simulink model "Rocket_test"  (R2019b)
settings: Solver=VariableStepAuto  StartTime=0  StopTime=100  FixedStep=0.001  MinStep=0.01  RelTol=1e-3
InitFcn:
  | initScript
undefined symbols (not defined in the file): aeng, Anoz, C_IE0, C_LE, cg_rocket, cg_total, Earth, J_rocket, J_total, K1_pitch, l_1st_stage, m_1st_stage_fuel, m_rocket, Omega_earth, Omega_I, P_pvp1, P_pvp2, P_pvp3, P_pvp4, r0, r_1st_stage, sim_dcm, traj_pitch, traj_t, traj_thrust, WGS84, x0, x_1st_stage
libraries: vrlib x9, sharedtransform x4, aerolibtransform2 x1, aerolibasang x1
settings Model: Creator=frizzer  LastModifiedBy=frizzer
settings SolverCC: ZeroCrossAlgorithm=Adaptive
settings DebuggingCC: IgnoredZcDiagnostic=none

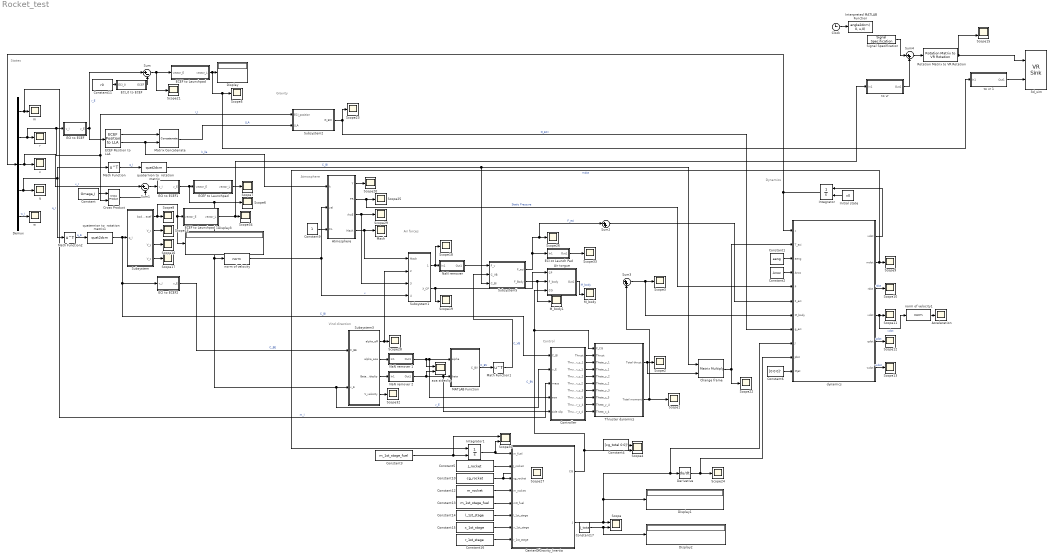
== system Rocket_test ==
  note: Dynamics
  note: Control
  note: Air forces
  note: Gravity
  note: States
  note: Atmosphere
  note: Vind direction
  "3d_sim " : vrlib/VR Sink  InstantiateOnLoad=on  SampleTime=0.1  ViewEnable=on  RemoteChange=off  RemoteView=on  FieldsWritten=Rocket.rotation.4.1.1.double#Rocket.translation.3.1.1.double  WorldFileName=rocket_test_vr.wrl  AutoView=off  VideoDimensions=[200 320]  AllowVariableSize=off  FigureProperties="{'Position', 'Name', 'Viewpoint', 'CameraBound', 'CameraDirection', 'CameraPosition', 'CameraUpVector', 'ZoomFactor', 'Antialiasing', 'Headlight', 'Lighting', 'NavPanel', 'Sound', 'StatusBar', 'Stereo3D', 'Stereo3DCameraOffset', 'Stereo3DHIT', 'ToolBar', 'Textures', 'Transparency', 'Triad', 'Wireframe', 'NavZones', 'NavMode', 'NavSpeed', 'CaptureFileFormat', 'CaptureFileName', 'Record2DCompressMethod', 'Record2DCompressQuality', 'Record2D', 'Record2DFileName', 'Record2DFPS'; [3.0850000000000000e+03   4.9600000000000000e+02   5.7600000000000000e+02   4.2900000000000000e+02], '', 'Rocket', 'on', [3.2020231009351967e-02   9.8606975468551894e-01  -1.6322114967293791e-01], [-4.4051406459118809e+01  -2.7334109397810590e+02  -6.6486808345328058e+01], [9.9894652123826644e-01  -3.6944163507175866e-02  -2.7220883319652722e-02], [1.0000000000000000e+00], 'off', 'on', 'on', 'halfbar', 'on', 'on', 'off', [1.0000000149011612e-01], [0.0000000000000000e+00], 'on', 'on', 'on', 'none', 'off', 'on', 'fly', 'veryslow', 'tif', '%f_anim_%n.tif', 'auto', [7.5000000000000000e+01], 'on', '%f_anim_%n.avi', 'auto'; [3.0000000000000000e+01   6.0000000000000000e+01   3.2000000000000000e+02   2.0000000000000000e+02], '', '', 'on', [0.0000000000000000e+00   0.0000000000000000e+00  -1.0000000000000000e+00], [0.0000000000000000e+00   0.0000000000000000e+00   7.2746134948730457e+01], [0.0000000000000000e+00   1.0000000000000000e+00   0.0000000000000000e+00], [1.0000000000000000e+00], 'on', 'on', 'on', 'none', 'on', 'off', 'off', [1.0000000149011612e-01], [0.0000000000000000e+00], 'off', 'on', 'on', 'none', 'off', 'off', 'fly', 'normal', 'tif', '%f_anim_%n.tif', 'auto', [7.5000000000000000e+01], 'off', '***video***', 'auto'}"
      settings: SourceProductName=Simulink
  "Acceleration " : Scope
  Air torgue : Subsystem
  Atmosphere : MATLAB Function  TreatAsAtomicUnit=on
  CenterOfGravity_Inertia : MATLAB Function  TreatAsAtomicUnit=on
  Change frame : Product  Multiplication=Matrix(*)
  Clock : Clock
  Constant : Constant  Value=Omega_I
  Constant1 : Constant  Value=aeng
  Constant10 : Constant  Value=cg_rocket
  Constant11 : Constant  Value=r0
  Constant12 : Constant  Value=m_rocket
  Constant13 : Constant  Value=m_1st_stage_fuel
  Constant14 : Constant  Value=l_1st_stage
  Constant15 : Constant  Value=x_1st_stage
  Constant16 : Constant  Value=r_1st_stage
  Constant17 : Constant  Value=J_total
  Constant2 : Constant  Value=Anoz
  Constant3 : Constant  Value=m_1st_stage_fuel
  Constant4 : Constant  Value=[cg_total 0 0]'
  Constant5 : Constant  Value=J_rocket
  Constant6 : Constant  Value=[0 0 0]'
  Constant9 : Constant
  Controller : Subsystem
  Cross Product : vrlib/Utilities/Cross Product
      settings: SourceProductName=Simulink
  Demux : Demux  Outputs=[1 3 3 4 3]
  Derivative : Derivative
  Display{,1..3} (4 alike) : Display
      Display settings: Decimation=6
      Display1 settings: Decimation=6
      Display2 settings: Decimation=6
  "ECEF Position to LLA " : aerolibtransform2/ECEF Position to LLA  units=Metric (MKS)  ptype=Earth (WGS84)  F=1/298.257223563  R=6378137
      settings: SourceProductName=Aerospace Blockset  SourceProductBaseCode=AE
  ECEF to Launchpad : Subsystem
  "ECEF to Launchpad " : Subsystem
  ECEF to Launchpad 1 : Subsystem
  ECI ot Launch Pad : Subsystem
  ECI to ECEF : Subsystem
  ECI to ECEF1 : Subsystem
  ECI to ECEF2 : Subsystem
  ECI_0 to ECEF : Subsystem
  Initial state : Constant  Value=x0
  Integrator : Integrator  InitialConditionSource=external  InitialCondition=x0
  Integrator1 : Integrator  InitialConditionSource=external  InitialCondition=x0
  Interpreted MATLAB Function : MATLABFcn  MATLABFcn=angle2dcm( 0, u,0)
  MATLAB Function : MATLAB Function  TreatAsAtomicUnit=on
  M_body : Scope
  M_body1 : Scope
  "Mach " : Scope
  Math Function : Math  Operator=transpose  SignedPower=off  SaturateOnIntegerOverflow=on
  Math Function1 : Math  Operator=transpose  SignedPower=off  SaturateOnIntegerOverflow=on
  Math Function2 : Math  Operator=transpose  SignedPower=off  SaturateOnIntegerOverflow=on
  Matrix Concatenate : Concatenate  ConcatenateDimension=3
  "NaN remover " : Subsystem
  NaN remover 1 : Subsystem
  NaN remover 2 : Subsystem
  Rotation Matrix to VR Rotation : vrlib/Utilities/Rotation Matrix to VR Rotation  maxzero=1e-12
      settings: SourceProductName=Simulink  SourceProductBaseCode=SL
  Scope{,4,15,30} (4 alike) : Scope  NumInputPorts=2
  Scope{1..3,5..14,16..29,32..34} (30 alike) : Scope
  Signal Specification : SignalSpecification  Dimensions=[3 3]
  Subsystem : Subsystem
  Subsystem1 : Subsystem
  Subsystem2 : Subsystem
  Subsystem3 : Subsystem
  Subsystem5 : Subsystem
  Sum : Sum  Inputs=|+-
  Sum1 : Sum  Inputs=|+-
  Sum2 : Sum  Inputs=|++
  Sum3 : Sum  Inputs=|++
  Sum4 : Sum  Inputs=|++
  Thruster dynamics : Subsystem
  "aoa sideslip " : Scope  NumInputPorts=2
  dynamics : MATLAB Function  TreatAsAtomicUnit=on
  m : Scope
  norm of velocity : MATLABFcn  MATLABFcn=norm  Output1D=off
  norm of velocity1 : MATLABFcn  MATLABFcn=norm  Output1D=off
  q : Scope
  quaternion to  rotation matrix : MATLABFcn  MATLABFcn=quat2dcm  Output1D=off
  quaternion to  rotation matrix1 : MATLABFcn  MATLABFcn=quat2dcm  Output1D=off
  r : Scope
  "to vr " : Subsystem
  to vr 1 : Subsystem
  v : Scope
  w : Scope
  wires:
  Initial state/1 -> Integrator/2
  Constant1/1 -> dynamics/3(aeng)
  ECEF to Launchpad/1(vector_L) -> Scope7/1
  dynamics/1(xdot) -> Integrator/1
  Sum2/1 -> dynamics/6(F_eci)
  Derivative/1 -> dynamics/10(Jdot), Scope24/1
  Constant11/1 -> ECI_0 to ECEF/1(ECI_0)
  Constant2/1 -> dynamics/4(Anoz)
  Constant/1 -> Cross Product/1
  dynamics/3(rdot) -> Scope10/1  "rdot"
  quaternion to  rotation matrix/1 -> Change frame/1, Subsystem5/3(C_BI)  "C_BI"
  Cross Product/1 -> Sum1/2
  dynamics/5(qdot) -> Scope12/1  "qdot"
  ECI to ECEF1/1(v_E) -> Controller/2(v_E), Subsystem3/2(v_E), norm of velocity/1, Scope6/1, ECEF to Launchpad/1("vector_E ")  "v_E"
  Subsystem5/1(F_eci) -> Sum2/1, Scope26/1, ECI ot Launch Pad/1(In1)  "F_eci"
  Sum1/1 -> ECI to ECEF1/1("v_I ")
  dynamics/6(wdot) -> Scope13/1  "wdot"
  ECI_0 to ECEF/1(ECEF) -> Sum/2
  Constant6/1 -> dynamics/11(Mjet)
  Subsystem/1(body in ecef) -> Display3/1, ECEF to Launchpad 1/1("vector_E "), Scope8/1
  dynamics/2(mdot) -> Integrator1/1, Scope9/1  "mdot"
  Math Function/1 -> quaternion to  rotation matrix/1  "q_I"
  Atmosphere/1(Y) -> Scope20/1
  Subsystem/4(V_z) -> Scope17/1
  Subsystem3/1(alpha_eff) -> Subsystem1/2(alpha_eff), Scope28/1
  ECI to ECEF2/1(v_E) -> Subsystem3/1(C_BE)  "C_BE"
  Subsystem3/4(V_velocity) -> Scope32/1
  Demux/4 -> q/1, Math Function/1, Math Function2/1  "q_I"
  Constant9/1 -> Atmosphere/3(CL)
  Subsystem3/2(alpha_aoa) -> NaN remover 1/1(In1)
  ECI ot Launch Pad/1(Out1) -> Scope33/1
  MATLAB Function/1(C_BV) -> Math Function1/1  "C_BV"
  Subsystem1/2("X_CP ") -> Scope19/1, Air torgue/1(CP)
  norm of velocity1/1 -> "Acceleration "/1
  Sum3/1 -> Scope3/1, dynamics/7(M_body)
  Atmosphere/3(rhoE) -> Subsystem1/3(air_density), Scope29/1
  Math Function1/1 -> Subsystem5/2(C_VB)  "C_VB"
  Air torgue/1(Out1) -> M_body/1  "M_body"
  Subsystem5/2(F_Body) -> M_body1/1, Air torgue/2(F_body)
  Subsystem3/3(Beta_sideslip) -> NaN remover 2/1(In1)
  Thruster dynamics/1(Total thrust) -> Change frame/2, Scope2/1
  quaternion to  rotation matrix1/1 -> ECI to ECEF2/1("v_I "), Controller/1(C_BI), Subsystem/1(q_I)  "C_BI"
  NaN remover 1/1(Out1) -> "aoa sideslip "/1, MATLAB Function/1(alpha), Controller/4(aoa)
  Change frame/1 -> dynamics/2(T_eci), Scope22/1
  Demux/1 -> Controller/3(mass), m/1  "m_I"
  Integrator/1 -> Demux/1, dynamics/1(x)
  CenterOfGravity_Inertia/2(J) -> Scope/1, dynamics/9(J), Derivative/1, Display1/1
  Atmosphere/2(PR) -> dynamics/5(P), Scope25/1  "Static Pressure"
  norm of velocity/1 -> Atmosphere/2(vel), Subsystem1/4(air_speed)  "v"
  Atmosphere/4(Mach) -> Subsystem1/1(Mach), "Mach "/1
  Subsystem1/1(F_aero) -> Scope18/1, "NaN remover "/1(In1)
  NaN remover 2/1(Out1) -> Controller/5(side slip), MATLAB Function/2(beta), "aoa sideslip "/2
  Thruster dynamics/2(Total moment) -> Sum3/2, Scope1/1
  Subsystem/2(V_x) -> Scope14/1
  dynamics/4(vdot) -> norm of velocity1/1, Scope11/1  "vdot"
  Matrix Concatenate/1 -> Subsystem2/2("LLA ")  "LLA"
  "NaN remover "/1(Out1) -> Subsystem5/1(F_v)
  Demux/5 -> w/1  "w_I"
  Math Function2/1 -> quaternion to  rotation matrix1/1  "q_E"
  Subsystem/3(V_y) -> Scope16/1
  "ECEF Position to LLA "/1 -> Matrix Concatenate/1
  Demux/2 -> r/1, Subsystem2/1(ECI_position), Cross Product/2, ECI to ECEF/1("v_I ")  "r_I"
  Demux/3 -> v/1, Sum1/1  "v_I"
  ECI to ECEF/1(v_E) -> "ECEF Position to LLA "/1, Sum/1  "r_E"
  "ECEF to Launchpad "/1(vector_L) -> to vr 1/1(In1), Scope5/1, Display/1
  Sum/1 -> "ECEF to Launchpad "/1("vector_E "), Scope21/1
  Subsystem2/1(G_ECI) -> Scope23/1, dynamics/8(g_eci)  "G_ECI"
  "ECEF Position to LLA "/2 -> Atmosphere/1(h), Matrix Concatenate/2  "h_lla"
  Constant3/1 -> Scope30/1, Integrator1/2
  Constant5/1 -> CenterOfGravity_Inertia/2(J_rocket)
  Constant10/1 -> Scope27/1, CenterOfGravity_Inertia/3(cg_rocket)
  Constant12/1 -> CenterOfGravity_Inertia/4(m_rocket)
  Constant13/1 -> CenterOfGravity_Inertia/5(m0_fuel)
  Constant14/1 -> CenterOfGravity_Inertia/6(l_1st_stage)
  Constant15/1 -> CenterOfGravity_Inertia/7(x_1st_stage)
  Constant16/1 -> CenterOfGravity_Inertia/8(r_1st_stage)
  CenterOfGravity_Inertia/1(CG) -> Thruster dynamics/1(P_CG), Air torgue/3(CG), Scope4/2  "C_BV"
  Constant17/1 -> Display2/1, Scope/2
  Integrator1/1 -> Scope30/2, CenterOfGravity_Inertia/1(m_fuel)
  Constant4/1 -> Scope4/1
  Controller/1(Thrust) -> Thruster dynamics/2(Thrust)
  Controller/2(Thruster_y_1) -> Thruster dynamics/3(Theta_y_1)
  Controller/3(Thruster_z_1) -> Thruster dynamics/4(Theta_z_1)
  Controller/4(Thruster_y_2) -> Thruster dynamics/5(Theta_y_2)
  Controller/5(Thruster_z_2) -> Thruster dynamics/6(Theta_z_2)
  Controller/6(Thruster_y_3) -> Thruster dynamics/7(Theta_y_3)
  Controller/7(Thruster_z_3) -> Thruster dynamics/8(Theta_z_3)
  Controller/8(Thruster_y_4) -> Thruster dynamics/9(Theta_y_4)
  Controller/9(Thruster_z_4) -> Thruster dynamics/10(Theta_z_4)
  Clock/1 -> Interpreted MATLAB Function/1
  Rotation Matrix to VR Rotation/1 -> Scope15/2, "3d_sim "/1
  ECEF to Launchpad 1/1(vector_L) -> "to vr "/1(In1), Scope34/1
  Signal Specification/1 -> Sum4/1
  Sum4/1 -> Rotation Matrix to VR Rotation/1
  "to vr "/1(Out1) -> Sum4/2
  to vr 1/1(Out1) -> "3d_sim "/2

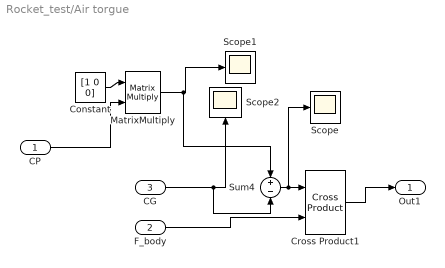
== system Rocket_test/Air torgue ==
  CP : Inport
  F_body : Inport  Port=2
  CG : Inport  Port=3
  Constant : Constant  Value=[1 0 0]
  Cross Product1 : vrlib/Utilities/Cross Product
      settings: SourceProductName=Simulink
  MatrixMultiply : Product  Multiplication=Matrix(*)
  Scope : Scope
  Scope1 : Scope
  Scope2 : Scope
  Sum4 : Sum  Inputs=+-
  Out1 : Outport
  wires:
  CP/1 -> MatrixMultiply/2
  Sum4/1 -> Scope/1, Cross Product1/1
  CG/1 -> Scope2/1, Sum4/2
  F_body/1 -> Cross Product1/2
  Cross Product1/1 -> Out1/1
  Constant/1 -> MatrixMultiply/1
  MatrixMultiply/1 -> Sum4/1, Scope1/1

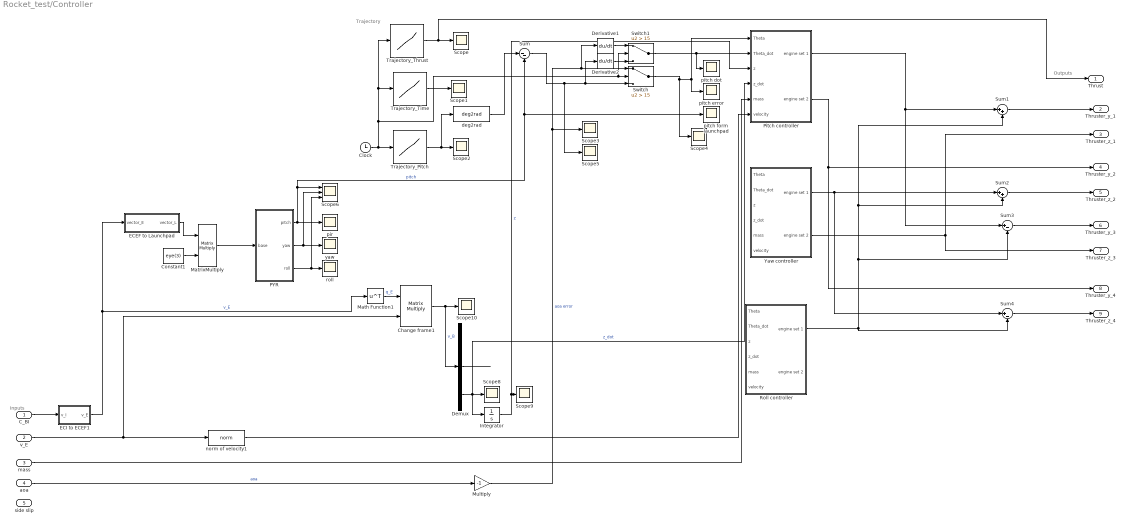
== system Rocket_test/Controller ==
  note: Inputs
  note: Trajectory
  note: Outputs
  C_BI : Inport
  v_E : Inport  Port=2
  mass : Inport  Port=3
  aoa : Inport  Port=4
  side slip : Inport  Port=5
  Change frame1 : Product  Multiplication=Matrix(*)
  Clock : Clock
  Constant1 : Constant  Value=eye(3)
  Demux : Demux  Outputs=3
  Derivative1 : Derivative
  Derivative2 : Derivative
  ECEF to Launchpad : Subsystem
  ECI to ECEF1 : Subsystem
  Integrator : Integrator
  Math Function1 : Math  Operator=transpose  SignedPower=off  SaturateOnIntegerOverflow=on
  MatrixMultiply : Product  Multiplication=Matrix(*)
  Multiply : Gain  Gain=-1
  PYR : MATLAB Function  TreatAsAtomicUnit=on
  Pitch controller : Subsystem
  Roll controller : Subsystem
  Scope{,1..5,8..10} (9 alike) : Scope
  Scope6 : Scope  NumInputPorts=3
  Sum : Sum  Inputs=|--
  Sum1 : Sum  Inputs=|++
  Sum2 : Sum  Inputs=|++
  Sum3 : Sum  Inputs=|+-
  Sum4 : Sum  Inputs=|+-
  Switch : Switch  Criteria=u2 > Threshold  Threshold=15
  Switch1 : Switch  Criteria=u2 > Threshold  Threshold=15
  Trajectory_Pitch : Lookup_n-D  NumberOfTableDimensions=1  BreakpointsForDimension1=traj_t  Table=traj_pitch  InternalRulePriority=Speed  RndMeth=Simplest  InputSameDT=on
  Trajectory_Thrust : Lookup_n-D  NumberOfTableDimensions=1  BreakpointsForDimension1=traj_t  Table=traj_thrust  InternalRulePriority=Speed  RndMeth=Simplest  InputSameDT=on
  Trajectory_Time : Lookup_n-D  NumberOfTableDimensions=1  BreakpointsForDimension1=traj_t  Table=traj_t  InternalRulePriority=Speed  RndMeth=Simplest  InputSameDT=on
  Yaw controller : Subsystem
  deg2rad : MATLABFcn  MATLABFcn=deg2rad
  norm of velocity1 : MATLABFcn  MATLABFcn=norm  Output1D=off
  pir : Scope
  pitch dot : Scope
  pitch error : Scope
  pitch form launchpad : Scope
  "roll " : Scope
  yaw : Scope
  Thrust : Outport
  Thruster_y_1 : Outport  Port=2
  Thruster_z_1 : Outport  Port=3
  Thruster_y_2 : Outport  Port=4
  Thruster_z_2 : Outport  Port=5
  Thruster_y_3 : Outport  Port=6
  Thruster_z_3 : Outport  Port=7
  Thruster_y_4 : Outport  Port=8
  Thruster_z_4 : Outport  Port=9
  wires:
  v_E/1 -> norm of velocity1/1, Change frame1/2
  norm of velocity1/1 -> Pitch controller/6(velocity)
  Change frame1/1 -> Scope10/1, Demux/1  "v_B"
  Math Function1/1 -> Change frame1/1  "q_E"
  deg2rad/1 -> Sum/1
  Roll controller/1(engine set 1) -> Sum4/2, Sum2/2, Sum1/2, Sum3/2
  MatrixMultiply/1 -> PYR/1(base)
  Yaw controller/1(engine set 1) -> Sum4/1, Sum2/1
  Sum4/1 -> Thruster_z_4/1
  C_BI/1 -> ECI to ECEF1/1("v_I ")
  Switch1/1 -> Pitch controller/2(Theta_dot), pitch dot/1
  Integrator/1 -> Pitch controller/3(z), Scope9/1  "z"
  Demux/3 -> Pitch controller/4(z_dot), Scope8/1, Integrator/1  "z_dot"
  Yaw controller/2(engine set 2) -> Thruster_z_3/1, Thruster_z_1/1
  Trajectory_Pitch/1 -> deg2rad/1, Scope2/1
  Pitch controller/1(engine set 1) -> Sum3/1, Sum1/1
  PYR/1(pitch) -> Sum/2, pitch form launchpad/1, Scope6/1, pir/1  "pitch"
  Sum3/1 -> Thruster_y_3/1
  Pitch controller/2(engine set 2) -> Thruster_y_4/1, Thruster_y_2/1
  ECI to ECEF1/1(v_E) -> ECEF to Launchpad/1("vector_E "), Math Function1/1  "v_E"
  mass/1 -> Pitch controller/5(mass)
  Clock/1 -> Switch1/2, Switch/2, Trajectory_Time/1, Trajectory_Thrust/1, Trajectory_Pitch/1
  PYR/2(yaw) -> yaw/1, Scope6/2
  ECEF to Launchpad/1(vector_L) -> MatrixMultiply/1
  Trajectory_Thrust/1 -> Thrust/1, Scope/1
  Constant1/1 -> MatrixMultiply/2
  PYR/3(roll) -> Scope6/3, "roll "/1
  Trajectory_Time/1 -> Scope1/1
  Sum2/1 -> Thruster_z_2/1
  Sum1/1 -> Thruster_y_1/1
  Demux/2 -> ?
  aoa/1 -> Multiply/1  "aoa"
  Sum/1 -> Scope5/1, Derivative2/1, Switch/3
  Switch/1 -> Pitch controller/1(Theta), pitch error/1, Scope4/1
  Derivative1/1 -> Switch1/1
  Derivative2/1 -> Switch1/3
  Multiply/1 -> Scope3/1, Derivative1/1, Switch/1  "aoa error"

== system Rocket_test/ECEF to Launchpad ==
  "vector_E " : Inport
  Change frame2 : Product  Multiplication=Matrix(*)
  ECEF to L 2 : Constant  Value=C_LE
  Math Function1 : Math  Operator=transpose  SignedPower=off  SaturateOnIntegerOverflow=on
  vector_L : Outport
  wires:
  "vector_E "/1 -> Change frame2/2
  ECEF to L 2/1 -> Math Function1/1
  Change frame2/1 -> vector_L/1
  Math Function1/1 -> Change frame2/1

== system Rocket_test/ECEF to Launchpad  ==
  "vector_E " : Inport
  Change frame2 : Product  Multiplication=Matrix(*)
  ECEF to L 2 : Constant  Value=C_LE
  Math Function1 : Math  Operator=transpose  SignedPower=off  SaturateOnIntegerOverflow=on
  vector_L : Outport
  wires:
  "vector_E "/1 -> Change frame2/2
  ECEF to L 2/1 -> Math Function1/1
  Change frame2/1 -> vector_L/1
  Math Function1/1 -> Change frame2/1

== system Rocket_test/ECEF to Launchpad 1 ==
  "vector_E " : Inport
  Change frame2 : Product  Multiplication=Matrix(*)
  ECEF to L 2 : Constant  Value=C_LE
  Math Function1 : Math  Operator=transpose  SignedPower=off  SaturateOnIntegerOverflow=on
  vector_L : Outport
  wires:
  "vector_E "/1 -> Change frame2/2
  ECEF to L 2/1 -> Math Function1/1
  Change frame2/1 -> vector_L/1
  Math Function1/1 -> Change frame2/1

== system Rocket_test/ECI ot Launch Pad ==
  In1 : Inport
  ECEF to Launchpad 1 : Subsystem
  ECI to ECEF4 : Subsystem
  Out1 : Outport
  wires:
  ECI to ECEF4/1(v_E) -> ECEF to Launchpad 1/1("vector_E ")
  ECEF to Launchpad 1/1(vector_L) -> Out1/1
  In1/1 -> ECI to ECEF4/1("v_I ")

== system Rocket_test/ECI to ECEF ==
  "v_I " : Inport
  Change frame2 : Product  Inputs=3  Multiplication=Matrix(*)
  Clock1 : Clock
  Constant1 : Constant  Value=Omega_earth
  ECEF to L 2 : Constant  Value=C_IE0
  MATLAB Function1 : MATLAB Function  TreatAsAtomicUnit=on
  v_E : Outport
  wires:
  MATLAB Function1/1(C_IE_t) -> Change frame2/1
  "v_I "/1 -> Change frame2/3
  Constant1/1 -> MATLAB Function1/2(Omega_earth)
  Clock1/1 -> MATLAB Function1/1(t)
  Change frame2/1 -> v_E/1
  ECEF to L 2/1 -> Change frame2/2

== system Rocket_test/ECI to ECEF1 ==
  "v_I " : Inport
  Change frame2 : Product  Inputs=3  Multiplication=Matrix(*)
  Clock1 : Clock
  Constant1 : Constant  Value=Omega_earth
  ECEF to L 2 : Constant  Value=C_IE0
  MATLAB Function1 : MATLAB Function  TreatAsAtomicUnit=on
  v_E : Outport
  wires:
  MATLAB Function1/1(C_IE_t) -> Change frame2/1
  "v_I "/1 -> Change frame2/3
  Constant1/1 -> MATLAB Function1/2(Omega_earth)
  Clock1/1 -> MATLAB Function1/1(t)
  Change frame2/1 -> v_E/1
  ECEF to L 2/1 -> Change frame2/2

== system Rocket_test/ECI to ECEF2 ==
  "v_I " : Inport
  Change frame2 : Product  Inputs=3  Multiplication=Matrix(*)
  Clock1 : Clock
  Constant1 : Constant  Value=Omega_earth
  ECEF to L 2 : Constant  Value=C_IE0
  MATLAB Function1 : MATLAB Function  TreatAsAtomicUnit=on
  v_E : Outport
  wires:
  ECEF to L 2/1 -> Change frame2/2
  Change frame2/1 -> v_E/1
  Clock1/1 -> MATLAB Function1/1(t)
  Constant1/1 -> MATLAB Function1/2(Omega_earth)
  "v_I "/1 -> Change frame2/3
  MATLAB Function1/1(C_IE_t) -> Change frame2/1

== system Rocket_test/ECI_0 to ECEF ==
  ECI_0 : Inport
  Constant12 : Constant  Value=C_IE0
  MatrixMultiply : Product  Multiplication=Matrix(*)
  ECEF : Outport
  wires:
  Constant12/1 -> MatrixMultiply/1
  MatrixMultiply/1 -> ECEF/1
  ECI_0/1 -> MatrixMultiply/2

== system Rocket_test/NaN remover  ==
  In1 : Inport
  Constant4 : Constant  Value=[0 0 0]'
  IsNaN : RelationalOperator  Operator=isNaN  OutDataTypeStr=boolean  RndMeth=Simplest
  "NaN " : Scope
  Switch : Switch  Criteria=u2 > Threshold
  Out1 : Outport
  wires:
  IsNaN/1 -> "NaN "/1, Switch/2
  Constant4/1 -> Switch/1
  In1/1 -> IsNaN/1, Switch/3
  Switch/1 -> Out1/1

== system Rocket_test/NaN remover 1 ==
  In1 : Inport
  Constant4 : Constant  Value=0
  IsNaN : RelationalOperator  Operator=isNaN  OutDataTypeStr=boolean  RndMeth=Simplest
  "NaN " : Scope
  Switch : Switch  Criteria=u2 > Threshold
  Out1 : Outport
  wires:
  Switch/1 -> Out1/1
  In1/1 -> Switch/3, IsNaN/1
  Constant4/1 -> Switch/1
  IsNaN/1 -> Switch/2, "NaN "/1

== system Rocket_test/NaN remover 2 ==
  In1 : Inport
  Constant4 : Constant  Value=0
  IsNaN : RelationalOperator  Operator=isNaN  OutDataTypeStr=boolean  RndMeth=Simplest
  "NaN " : Scope
  Switch : Switch  Criteria=u2 > Threshold
  Out1 : Outport
  wires:
  IsNaN/1 -> "NaN "/1, Switch/2
  Constant4/1 -> Switch/1
  In1/1 -> IsNaN/1, Switch/3
  Switch/1 -> Out1/1

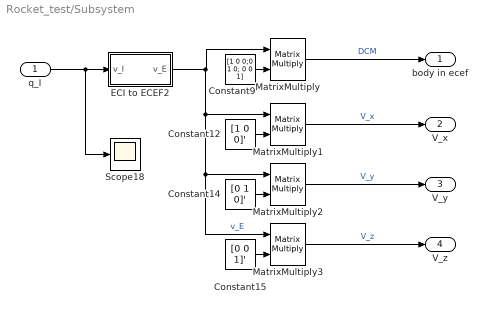
== system Rocket_test/Subsystem ==
  q_I : Inport
  Constant12 : Constant  Value=[1 0 0]'
  Constant14 : Constant  Value=[0 1 0]'
  Constant15 : Constant  Value=[0 0 1]'
  Constant9 : Constant  Value=[1 0 0;0 1 0; 0 0 1]
  ECI to ECEF2 : Subsystem
  MatrixMultiply{,1..3} (4 alike) : Product  Multiplication=Matrix(*)
  Scope18 : Scope
  body in ecef : Outport
  V_x : Outport  Port=2
  V_y : Outport  Port=3
  V_z : Outport  Port=4
  wires:
  MatrixMultiply/1 -> body in ecef/1  "DCM"
  ECI to ECEF2/1(v_E) -> MatrixMultiply3/1, MatrixMultiply2/1, MatrixMultiply1/1, MatrixMultiply/1  "v_E"
  q_I/1 -> Scope18/1, ECI to ECEF2/1("v_I ")
  Constant9/1 -> MatrixMultiply/2
  Constant14/1 -> MatrixMultiply2/2
  Constant12/1 -> MatrixMultiply1/2
  MatrixMultiply1/1 -> V_x/1  "V_x"
  Constant15/1 -> MatrixMultiply3/2
  MatrixMultiply2/1 -> V_y/1  "V_y"
  MatrixMultiply3/1 -> V_z/1  "V_z"

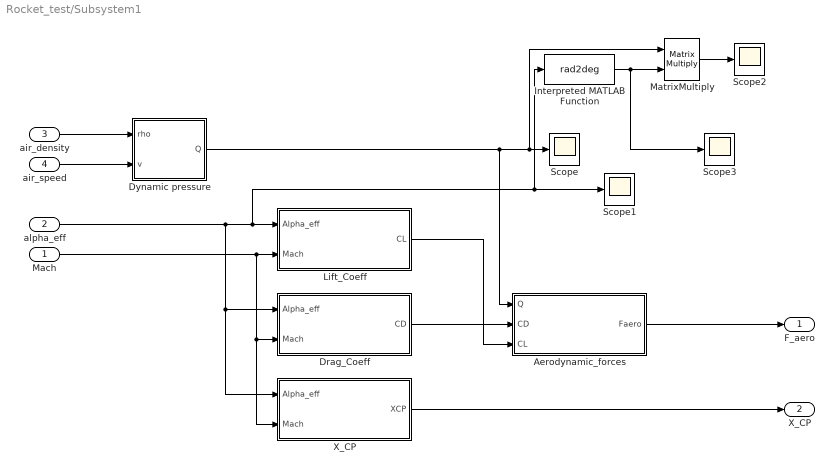
== system Rocket_test/Subsystem1 ==
  Mach : Inport
  alpha_eff : Inport  Port=2
  air_density : Inport  Port=3
  air_speed : Inport  Port=4
  Aerodynamic_forces : MATLAB Function  TreatAsAtomicUnit=on
  Drag_Coeff : MATLAB Function  TreatAsAtomicUnit=on
  Dynamic pressure : MATLAB Function  TreatAsAtomicUnit=on
  Interpreted MATLAB Function : MATLABFcn  MATLABFcn=rad2deg
  Lift_Coeff : MATLAB Function  TreatAsAtomicUnit=on
  MatrixMultiply : Product  Multiplication=Matrix(*)
  Scope{,1..3} (4 alike) : Scope
  X_CP : MATLAB Function  TreatAsAtomicUnit=on
  F_aero : Outport
  "X_CP " : Outport  Port=2
  wires:
  air_density/1 -> Dynamic pressure/1(rho)
  X_CP/1(XCP) -> "X_CP "/1
  Mach/1 -> X_CP/2(Mach), Drag_Coeff/2(Mach), Lift_Coeff/2(Mach)
  Lift_Coeff/1(CL) -> Aerodynamic_forces/3(CL)
  Drag_Coeff/1(CD) -> Aerodynamic_forces/2(CD)
  Aerodynamic_forces/1(Faero) -> F_aero/1
  alpha_eff/1 -> X_CP/1(Alpha_eff), Drag_Coeff/1(Alpha_eff), Interpreted MATLAB Function/1, Scope1/1, Lift_Coeff/1(Alpha_eff)
  Dynamic pressure/1(Q) -> MatrixMultiply/1, Scope/1, Aerodynamic_forces/1(Q)
  air_speed/1 -> Dynamic pressure/2(v)
  MatrixMultiply/1 -> Scope2/1
  Interpreted MATLAB Function/1 -> Scope3/1, MatrixMultiply/2

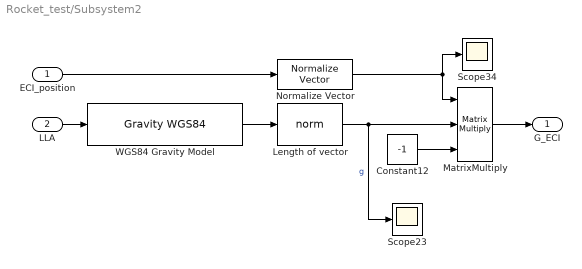
== system Rocket_test/Subsystem2 ==
  ECI_position : Inport
  "LLA " : Inport  Port=2
  Constant12 : Constant  Value=-1
  Length of vector : MATLABFcn  MATLABFcn=norm  Output1D=off
  MatrixMultiply : Product  Inputs=3  Multiplication=Matrix(*)
  Normalize Vector : vrlib/Utilities/Normalize Vector  maxzero=0
      settings: SourceProductName=Simulink
  Scope23 : Scope
  Scope34 : Scope
  "WGS84 Gravity Model  " : GravityWGS84  BlockKeywords=__PRM__SERIALIZED__DATA__:world geodetic system,WGS 84,geocentric,equipotential,ellipsoid,WGS84 taylor series,WGS84 close approximation,WGS84 exact,Earth,1984,Earth gravity,planetary gravity,gravitational field
  G_ECI : Outport
  wires:
  Length of vector/1 -> Scope23/1, MatrixMultiply/2  "g"
  Normalize Vector/1 -> MatrixMultiply/1, Scope34/1
  MatrixMultiply/1 -> G_ECI/1
  "WGS84 Gravity Model  "/1 -> Length of vector/1
  Constant12/1 -> MatrixMultiply/3
  "LLA "/1 -> "WGS84 Gravity Model  "/1
  ECI_position/1 -> Normalize Vector/1

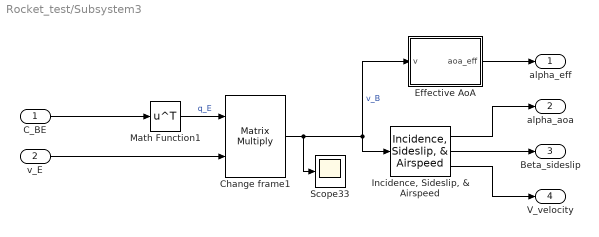
== system Rocket_test/Subsystem3 ==
  C_BE : Inport
  v_E : Inport  Port=2
  Change frame1 : Product  Multiplication=Matrix(*)
  Effective AoA : MATLAB Function  TreatAsAtomicUnit=on
  "Incidence, Sideslip, & Airspeed" : aerolibasang/Incidence, Sideslip, & Airspeed
      settings: SourceProductName=Aerospace Blockset
  Math Function1 : Math  Operator=transpose  SignedPower=off  SaturateOnIntegerOverflow=on
  Scope33 : Scope
  alpha_eff : Outport
  alpha_aoa : Outport  Port=2
  Beta_sideslip : Outport  Port=3
  V_velocity : Outport  Port=4
  wires:
  "Incidence, Sideslip, & Airspeed"/3 -> V_velocity/1
  Math Function1/1 -> Change frame1/1  "q_E"
  Change frame1/1 -> Scope33/1, Effective AoA/1(v), "Incidence, Sideslip, & Airspeed"/1  "v_B"
  C_BE/1 -> Math Function1/1
  Effective AoA/1(aoa_eff) -> alpha_eff/1
  v_E/1 -> Change frame1/2
  "Incidence, Sideslip, & Airspeed"/1 -> alpha_aoa/1
  "Incidence, Sideslip, & Airspeed"/2 -> Beta_sideslip/1

== system Rocket_test/Subsystem5 ==
  F_v : Inport
  C_VB : Inport  Port=2
  C_BI : Inport  Port=3
  MatrixMultiply : Product  Multiplication=Matrix(*)
  MatrixMultiply1 : Product  Multiplication=Matrix(*)
  F_eci : Outport
  F_Body : Outport  Port=2
  wires:
  F_v/1 -> MatrixMultiply/2
  MatrixMultiply/1 -> F_Body/1, MatrixMultiply1/2
  C_VB/1 -> MatrixMultiply/1
  C_BI/1 -> MatrixMultiply1/1
  MatrixMultiply1/1 -> F_eci/1

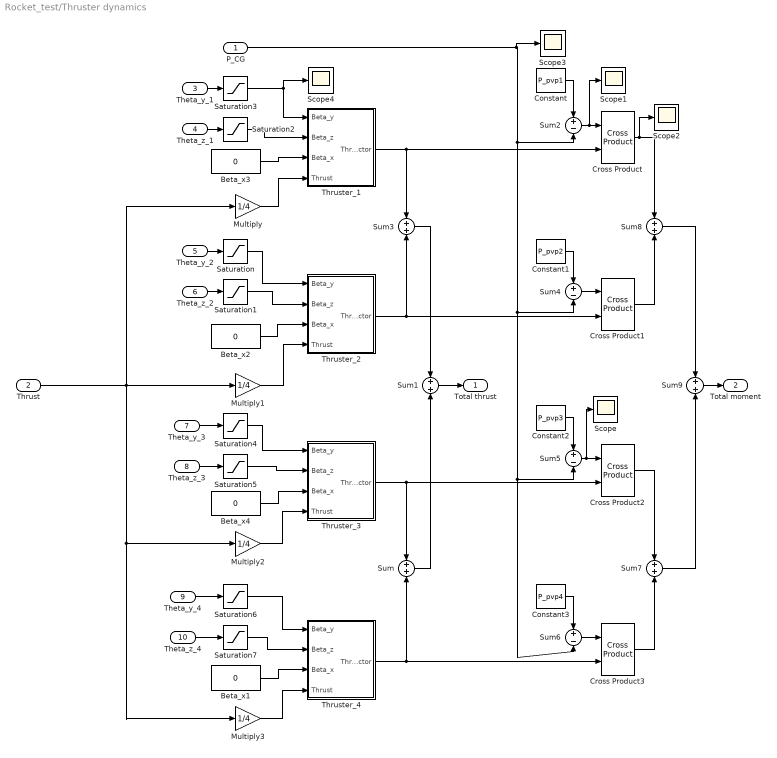
== system Rocket_test/Thruster dynamics ==
  P_CG : Inport
  Thrust : Inport  Port=2
  Theta_y_1 : Inport  Port=3
  Theta_z_1 : Inport  Port=4
  Theta_y_2 : Inport  Port=5
  Theta_z_2 : Inport  Port=6
  Theta_y_3 : Inport  Port=7
  Theta_z_3 : Inport  Port=8
  Theta_y_4 : Inport  Port=9
  Theta_z_4 : Inport  Port=10
  Beta_x{1..4} (4 alike) : Constant  Value=0
  Constant : Constant  Value=P_pvp1
  Constant1 : Constant  Value=P_pvp2
  Constant2 : Constant  Value=P_pvp3
  Constant3 : Constant  Value=P_pvp4
  Cross Product{,1..3} (4 alike) : vrlib/Utilities/Cross Product
      settings: SourceProductName=Simulink
  Multiply{,1..3} (4 alike) : Gain  Gain=1/4
  Saturation : Saturate  UpperLimit=deg2rad(6)  LowerLimit=deg2rad(-6)
  Saturation{1..7} (7 alike) : Saturate  UpperLimit=deg2rad(6)  LowerLimit=deg2rad(-6)  ZeroCross=off
  Scope{,1..4} (5 alike) : Scope
  Sum{,1,3,7..9} (6 alike) : Sum
  Sum{2,4..6} (4 alike) : Sum  Inputs=+-
  Thruster_1 : Subsystem
  Thruster_2 : Subsystem
  Thruster_3 : Subsystem
  Thruster_4 : Subsystem
  Total thrust : Outport
  Total moment : Outport  Port=2
  wires:
  Thrust/1 -> Multiply3/1, Multiply2/1, Multiply1/1, Multiply/1
  Beta_x1/1 -> Thruster_4/3(Beta_x)
  Theta_z_4/1 -> Saturation7/1
  Theta_y_4/1 -> Saturation6/1
  Thruster_4/1(Thrust_vector) -> Sum/2, Cross Product3/2
  Theta_y_3/1 -> Saturation4/1
  Theta_z_3/1 -> Saturation5/1
  Beta_x4/1 -> Thruster_3/3(Beta_x)
  Thruster_3/1(Thrust_vector) -> Cross Product2/2, Sum/1
  Thruster_1/1(Thrust_vector) -> Cross Product/2, Sum3/1
  Beta_x3/1 -> Thruster_1/3(Beta_x)
  Theta_z_1/1 -> Saturation2/1
  Theta_y_1/1 -> Saturation3/1
  Thruster_2/1(Thrust_vector) -> Sum3/2, Cross Product1/2
  Theta_y_2/1 -> Saturation/1
  Theta_z_2/1 -> Saturation1/1
  Beta_x2/1 -> Thruster_2/3(Beta_x)
  Sum3/1 -> Sum1/1
  Sum/1 -> Sum1/2
  Sum1/1 -> Total thrust/1
  P_CG/1 -> Scope3/1, Sum2/2, Sum4/2, Sum5/2, Sum6/2
  Sum2/1 -> Scope1/1, Cross Product/1
  Constant/1 -> Sum2/1
  Constant1/1 -> Sum4/1
  Sum4/1 -> Cross Product1/1
  Sum5/1 -> Scope/1, Cross Product2/1
  Constant2/1 -> Sum5/1
  Constant3/1 -> Sum6/1
  Sum6/1 -> Cross Product3/1
  Cross Product3/1 -> Sum7/2
  Cross Product2/1 -> Sum7/1
  Cross Product1/1 -> Sum8/2
  Cross Product/1 -> Scope2/1, Sum8/1
  Sum8/1 -> Sum9/1
  Sum7/1 -> Sum9/2
  Sum9/1 -> Total moment/1
  Multiply/1 -> Thruster_1/4(Thrust)
  Multiply1/1 -> Thruster_2/4(Thrust)
  Multiply2/1 -> Thruster_3/4(Thrust)
  Multiply3/1 -> Thruster_4/4(Thrust)
  Saturation/1 -> Thruster_2/1(Beta_y)
  Saturation1/1 -> Thruster_2/2(Beta_z)
  Saturation2/1 -> Thruster_1/2(Beta_z)
  Saturation3/1 -> Scope4/1, Thruster_1/1(Beta_y)
  Saturation4/1 -> Thruster_3/1(Beta_y)
  Saturation5/1 -> Thruster_3/2(Beta_z)
  Saturation6/1 -> Thruster_4/1(Beta_y)
  Saturation7/1 -> Thruster_4/2(Beta_z)

== system Rocket_test/to vr  ==
  In1 : Inport
  Constant7 : Constant  Value=sim_dcm
  MatrixMultiply : Product  Multiplication=Matrix(*)
  Out1 : Outport
  wires:
  Constant7/1 -> MatrixMultiply/1
  MatrixMultiply/1 -> Out1/1
  In1/1 -> MatrixMultiply/2

== system Rocket_test/to vr 1 ==
  In1 : Inport
  Constant7 : Constant  Value=sim_dcm
  MatrixMultiply : Product  Multiplication=Matrix(*)
  Out1 : Outport
  wires:
  In1/1 -> MatrixMultiply/2
  MatrixMultiply/1 -> Out1/1
  Constant7/1 -> MatrixMultiply/1

== system Rocket_test/Controller/ECEF to Launchpad ==
  "vector_E " : Inport
  Change frame2 : Product  Multiplication=Matrix(*)
  ECEF to L 2 : Constant  Value=C_LE
  Math Function1 : Math  Operator=transpose  SignedPower=off  SaturateOnIntegerOverflow=on
  vector_L : Outport
  wires:
  "vector_E "/1 -> Change frame2/2
  ECEF to L 2/1 -> Math Function1/1
  Change frame2/1 -> vector_L/1
  Math Function1/1 -> Change frame2/1

== system Rocket_test/Controller/ECI to ECEF1 ==
  "v_I " : Inport
  Change frame2 : Product  Inputs=3  Multiplication=Matrix(*)
  Clock1 : Clock
  Constant1 : Constant  Value=Omega_earth
  ECEF to L 2 : Constant  Value=C_IE0
  MATLAB Function1 : MATLAB Function  TreatAsAtomicUnit=on
  v_E : Outport
  wires:
  MATLAB Function1/1(C_IE_t) -> Change frame2/1
  "v_I "/1 -> Change frame2/3
  Constant1/1 -> MATLAB Function1/2(Omega_earth)
  Clock1/1 -> MATLAB Function1/1(t)
  Change frame2/1 -> v_E/1
  ECEF to L 2/1 -> Change frame2/2

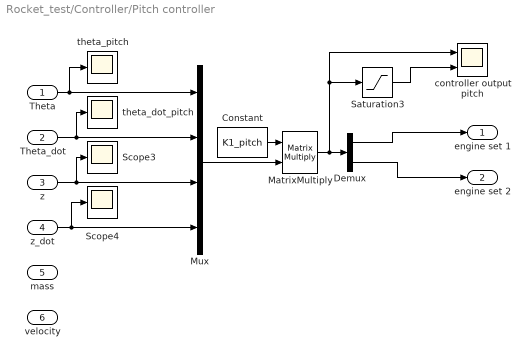
== system Rocket_test/Controller/Pitch controller ==
  Theta : Inport
  Theta_dot : Inport  Port=2
  z : Inport  Port=3
  z_dot : Inport  Port=4
  mass : Inport  Port=5
  velocity : Inport  Port=6
  Constant : Constant  Value=K1_pitch  VectorParams1D=off
  Demux : Demux  Outputs=2
  MatrixMultiply : Product  Multiplication=Matrix(*)
  Mux : Mux
  Saturation3 : Saturate  UpperLimit=deg2rad(6)  LowerLimit=deg2rad(-6)  LinearizeAsGain=off  ZeroCross=off
  Scope3 : Scope
  Scope4 : Scope
  controller output pitch : Scope  NumInputPorts=2
  theta_dot_pitch : Scope
  theta_pitch : Scope
  engine set 1 : Outport
  engine set 2 : Outport  Port=2
  wires:
  Demux/2 -> engine set 2/1
  z_dot/1 -> Scope4/1, Mux/4
  Demux/1 -> engine set 1/1
  Mux/1 -> MatrixMultiply/2
  Theta/1 -> theta_pitch/1, Mux/1
  MatrixMultiply/1 -> Saturation3/1, controller output pitch/1, Demux/1
  Constant/1 -> MatrixMultiply/1
  Theta_dot/1 -> theta_dot_pitch/1, Mux/2
  z/1 -> Scope3/1, Mux/3
  Saturation3/1 -> controller output pitch/2

== system Rocket_test/Controller/Roll controller ==
  Theta : Inport
  Theta_dot : Inport  Port=2
  z : Inport  Port=3
  z_dot : Inport  Port=4
  mass : Inport  Port=5
  velocity : Inport  Port=6
  engine set 1 : Outport
  engine set 2 : Outport  Port=2

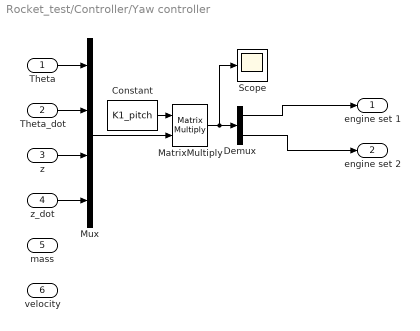
== system Rocket_test/Controller/Yaw controller ==
  Theta : Inport
  Theta_dot : Inport  Port=2
  z : Inport  Port=3
  z_dot : Inport  Port=4
  mass : Inport  Port=5
  velocity : Inport  Port=6
  Constant : Constant  Value=K1_pitch  VectorParams1D=off
  Demux : Demux  Outputs=2
  MatrixMultiply : Product  Multiplication=Matrix(*)
  Mux : Mux
  Scope : Scope
  engine set 1 : Outport
  engine set 2 : Outport  Port=2
  wires:
  z_dot/1 -> Mux/4
  z/1 -> Mux/3
  Theta_dot/1 -> Mux/2
  Theta/1 -> Mux/1
  Mux/1 -> MatrixMultiply/2
  Constant/1 -> MatrixMultiply/1
  MatrixMultiply/1 -> Scope/1, Demux/1
  Demux/1 -> engine set 1/1
  Demux/2 -> engine set 2/1

== system Rocket_test/ECI ot Launch Pad/ECEF to Launchpad 1 ==
  "vector_E " : Inport
  Change frame2 : Product  Multiplication=Matrix(*)
  ECEF to L 2 : Constant  Value=C_LE
  Math Function1 : Math  Operator=transpose  SignedPower=off  SaturateOnIntegerOverflow=on
  vector_L : Outport
  wires:
  Math Function1/1 -> Change frame2/1
  Change frame2/1 -> vector_L/1
  ECEF to L 2/1 -> Math Function1/1
  "vector_E "/1 -> Change frame2/2

== system Rocket_test/ECI ot Launch Pad/ECI to ECEF4 ==
  "v_I " : Inport
  Change frame2 : Product  Inputs=3  Multiplication=Matrix(*)
  Clock1 : Clock
  Constant1 : Constant  Value=Omega_earth
  ECEF to L 2 : Constant  Value=C_IE0
  MATLAB Function1 : MATLAB Function  TreatAsAtomicUnit=on
  v_E : Outport
  wires:
  ECEF to L 2/1 -> Change frame2/2
  Change frame2/1 -> v_E/1
  Clock1/1 -> MATLAB Function1/1(t)
  Constant1/1 -> MATLAB Function1/2(Omega_earth)
  "v_I "/1 -> Change frame2/3
  MATLAB Function1/1(C_IE_t) -> Change frame2/1

== system Rocket_test/Subsystem/ECI to ECEF2 ==
  "v_I " : Inport
  Change frame2 : Product  Inputs=3  Multiplication=Matrix(*)
  Clock1 : Clock
  Constant1 : Constant  Value=Omega_earth
  ECEF to L 2 : Constant  Value=C_IE0
  MATLAB Function1 : MATLAB Function  TreatAsAtomicUnit=on
  Transpose : Math  Operator=transpose  SignedPower=off  SaturateOnIntegerOverflow=on
  v_E : Outport
  wires:
  ECEF to L 2/1 -> Change frame2/2
  Change frame2/1 -> v_E/1
  Clock1/1 -> MATLAB Function1/1(t)
  Constant1/1 -> MATLAB Function1/2(Omega_earth)
  "v_I "/1 -> Change frame2/3
  MATLAB Function1/1(C_IE_t) -> Transpose/1
  Transpose/1 -> Change frame2/1

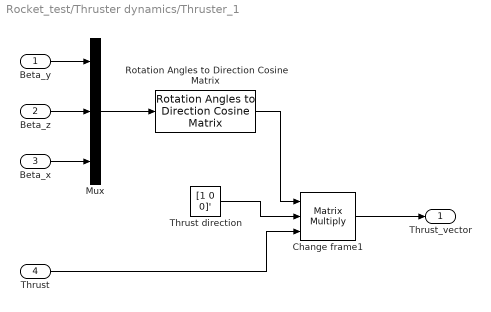
== system Rocket_test/Thruster dynamics/Thruster_1 ==
  Beta_y : Inport
  Beta_z : Inport  Port=2
  Beta_x : Inport  Port=3
  Thrust : Inport  Port=4
  Change frame1 : Product  Inputs=3  Multiplication=Matrix(*)
  Mux : Mux  Inputs=3
  Rotation Angles to Direction Cosine Matrix : sharedtransform/Rotation Angles to Direction Cosine Matrix  rotationOrder=YZX  aMode=aMode
      settings: SourceProductBaseCode=AE
  Thrust direction : Constant  Value=[1 0 0]'
  Thrust_vector : Outport
  wires:
  Change frame1/1 -> Thrust_vector/1
  Beta_y/1 -> Mux/1
  Beta_z/1 -> Mux/2
  Rotation Angles to Direction Cosine Matrix/1 -> Change frame1/1
  Thrust direction/1 -> Change frame1/2
  Beta_x/1 -> Mux/3
  Thrust/1 -> Change frame1/3
  Mux/1 -> Rotation Angles to Direction Cosine Matrix/1

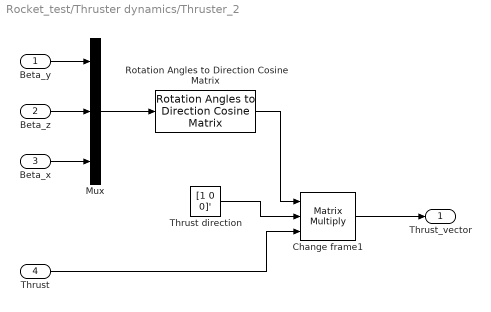
== system Rocket_test/Thruster dynamics/Thruster_2 ==
  Beta_y : Inport
  Beta_z : Inport  Port=2
  Beta_x : Inport  Port=3
  Thrust : Inport  Port=4
  Change frame1 : Product  Inputs=3  Multiplication=Matrix(*)
  Mux : Mux  Inputs=3
  Rotation Angles to Direction Cosine Matrix : sharedtransform/Rotation Angles to Direction Cosine Matrix  rotationOrder=YZX  aMode=aMode
      settings: SourceProductBaseCode=AE
  Thrust direction : Constant  Value=[1 0 0]'
  Thrust_vector : Outport
  wires:
  Mux/1 -> Rotation Angles to Direction Cosine Matrix/1
  Thrust/1 -> Change frame1/3
  Beta_x/1 -> Mux/3
  Thrust direction/1 -> Change frame1/2
  Rotation Angles to Direction Cosine Matrix/1 -> Change frame1/1
  Beta_z/1 -> Mux/2
  Beta_y/1 -> Mux/1
  Change frame1/1 -> Thrust_vector/1

== system Rocket_test/Thruster dynamics/Thruster_3 ==
  Beta_y : Inport
  Beta_z : Inport  Port=2
  Beta_x : Inport  Port=3
  Thrust : Inport  Port=4
  Change frame1 : Product  Inputs=3  Multiplication=Matrix(*)
  Mux : Mux  Inputs=3
  Rotation Angles to Direction Cosine Matrix : sharedtransform/Rotation Angles to Direction Cosine Matrix  rotationOrder=YZX  aMode=aMode
      settings: SourceProductBaseCode=AE
  Thrust direction : Constant  Value=[1 0 0]'
  Thrust_vector : Outport
  wires:
  Mux/1 -> Rotation Angles to Direction Cosine Matrix/1
  Thrust/1 -> Change frame1/3
  Beta_x/1 -> Mux/3
  Thrust direction/1 -> Change frame1/2
  Rotation Angles to Direction Cosine Matrix/1 -> Change frame1/1
  Beta_z/1 -> Mux/2
  Beta_y/1 -> Mux/1
  Change frame1/1 -> Thrust_vector/1

== system Rocket_test/Thruster dynamics/Thruster_4 ==
  Beta_y : Inport
  Beta_z : Inport  Port=2
  Beta_x : Inport  Port=3
  Thrust : Inport  Port=4
  Change frame1 : Product  Inputs=3  Multiplication=Matrix(*)
  Mux : Mux  Inputs=3
  Rotation Angles to Direction Cosine Matrix : sharedtransform/Rotation Angles to Direction Cosine Matrix  rotationOrder=YZX  aMode=aMode
      settings: SourceProductBaseCode=AE
  Thrust direction : Constant  Value=[1 0 0]'
  Thrust_vector : Outport
  wires:
  Change frame1/1 -> Thrust_vector/1
  Beta_y/1 -> Mux/1
  Beta_z/1 -> Mux/2
  Rotation Angles to Direction Cosine Matrix/1 -> Change frame1/1
  Thrust direction/1 -> Change frame1/2
  Beta_x/1 -> Mux/3
  Thrust/1 -> Change frame1/3
  Mux/1 -> Rotation Angles to Direction Cosine Matrix/1

== matlab function Rocket_test/Subsystem/ECI to ECEF2/MATLAB Function1 ==
  data: t input; C_IE_t output; Omega_earth input
function C_IE_t=ECI2ECEF(t,Omega_earth)
   C_IE_t =  [cos(Omega_earth*t)     sin(Omega_earth*t)  0;...
             -sin(Omega_earth*t)    cos(Omega_earth*t)  0;...
             0                      0                   1];
end

== matlab function Rocket_test/dynamics ==
  data: x input; xdot output; T_eci input; aeng input; Anoz input; P input; F_eci input; M_body input; g_eci input; J input; Jdot input; Mjet input; mdot output; rdot output; vdot output; qdot output; wdot output
function [xdot, mdot, rdot, vdot, qdot, wdot] = dynamics(x,T_eci,aeng,Anoz,P,F_eci,M_body,g_eci,J,Jdot,Mjet)

% INPUTS
% x      - state vector
% T_eci  - thrust force in ECI frame
% aeng   - mass depletion constant (Isp*g0)^-1
% Anoz   - engine nozzle area
% P      - atmospheric pressure
% F_eci  - sum of non-propulsive forces in ECI frame
% M_body - sum of moments in body frame
% g_eci  - gravity acceleration in ECI frame
% J      - inertia matrix
% Jdot   - inertia matrix derivative
% Mjet   - engine jet damping moment

% State vector
m=x(1);
r=x(2:4);
v=x(5:7);
q=x(8:11);
w=x(12:14);

% Propulsion
T=norm(T_eci);
mdot=-aeng*(T+P*Anoz);

% Translational ECI
F=T_eci+F_eci+m*g_eci;
vdot=F/m;
rdot=v;

% Quaternions
qdot=1/2*[q(4) -q(3)  q(2);
          q(3)  q(4) -q(1);
         -q(2)  q(1)  q(4);
         -q(1) -q(2) -q(3)]*w;

% Rotational BODY
M=M_body-Mjet-Jdot*w;
wdot=J\(-sksim(w)*J*w+M);

% State derivative -> to be integrated
xdot=[mdot;rdot;vdot;qdot;wdot];

end


function M=sksim(w)

M=[   0 -w(3) w(2);
    w(3)   0 -w(1);
   -w(2) w(1)   0];

end

== matlab function Rocket_test/ECI to ECEF/MATLAB Function1 ==
  data: t input; C_IE_t output; Omega_earth input
function C_IE_t=ECI2ECEF(t,Omega_earth)
   C_IE_t =  [cos(Omega_earth*t)     sin(Omega_earth*t)  0;...
             -sin(Omega_earth*t)    cos(Omega_earth*t)  0;...
             0                      0                   1];
end

== matlab function Rocket_test/ECI to ECEF1/MATLAB Function1 ==
  data: t input; C_IE_t output; Omega_earth input
function C_IE_t=ECI2ECEF(t,Omega_earth)
   C_IE_t =  [cos(Omega_earth*t)     sin(Omega_earth*t)  0;...
             -sin(Omega_earth*t)    cos(Omega_earth*t)  0;...
             0                      0                   1];
end

== matlab function Rocket_test/CenterOfGravity_Inertia ==
  data: m_fuel input; CG output; J_rocket input; cg_rocket input; m_rocket input; m0_fuel input; l_1st_stage input; x_1st_stage input; r_1st_stage input; J output
function [CG,J] = Center_Gravitation(m_fuel, J_rocket, cg_rocket, m_rocket, m0_fuel, l_1st_stage, x_1st_stage, r_1st_stage)
%Cg_r is the center of gravitation of the rocket.
%m_r is the mass of the rocket without fuel
%Cg_f is the center of gravitation of the fuel
%m_f is the mass of the fuel
%J is the inertia
%M is the total mass of the rocket and the fuel

m_procent_fuel=m_fuel/m0_fuel; % procent of max fuel

l_fuel= l_1st_stage*m_procent_fuel; %length of fuel

cg_1st_stage_fuel=(x_1st_stage)+(l_fuel)/(2)%make variable
CG_x=(m_rocket*cg_rocket+m_fuel*cg_1st_stage_fuel)/(m_rocket+m_fuel);
d_fuel=abs(cg_1st_stage_fuel-CG_x);
Jx_fuel=0.5*m_fuel*r_1st_stage^2;

Jyz_fuel=1/4*m_fuel*r_1st_stage^2+1/12*m_fuel...
    *l_fuel^2+m_fuel*d_fuel^2;



J_fuel = diag([Jx_fuel,Jyz_fuel,Jyz_fuel]);
J=J_fuel+J_rocket;
CG=[CG_x 0 0]';


    return;
end

== matlab function Rocket_test/Subsystem1/Lift_Coeff ==
  data: Alpha_eff input; CL output; Mach input
function CL = Lift_Coeff(Alpha_eff ,Mach)



CL = (Alpha_eff * 0.04) * (1 + Mach/4);
    return;
end

== matlab function Rocket_test/Atmosphere ==
  data: h input; Y output; vel input; CL input; PR output; rhoE output; Mach output
function [Y,PR,rhoE,Mach] = atmosphere(h, vel, CL)
%(c) 2005 Ashish Tewari
Y=zeros(10,1);
PR=0;
Mach=0;
rhoE=0;
R = 287; %sea-level gas constant for air (J/kg.K)
go = 9.806; %sea level acceleration due to gravity (m/s^2)
Na = 6.0220978e23; %Avogadro’s number
sigma = 3.65e-10; %collision diameter (m) for air
S = 110.4; %Sutherland’s temperature (K)
Mo = 28.964; %sea level molecular weight (g/mole)
To = 288.15; %sea level temperature (K)
Po = 1.01325e5; %sea level pressure (N/m^2)
re = 6378.14e3; %earth’s mean radius (m)
Beta = 1.458e-6; %Sutherland’s constant (kg/m.s.K^0.5)
gamma = 1.405; %sea level specific-heat ratio
B = 2/re; layers = 21; Z = 1e3*[0.00; 11.0191; 20.0631; 32.1619;
    47.3501; 51.4125;
    71.8020; 86.00; 100.00; 110.00; 120.00; 150.00; 160.00; 170.00; 190.00;
    230.00; 300.00; 400.00; 500.00; 600.00; 700.00; 2000.00];
T = [To; 216.65; 216.65; 228.65; 270.65; 270.65; 214.65; 186.946;
    210.65; 260.65; 360.65; 960.65; 1110.60; 1210.65; 1350.65; 1550.65;
    1830.65; 2160.65; 2420.65; 2590.65; 2700.00; 2700.0];
M = [Mo; 28.964; 28.964; 28.964; 28.964; 28.964; 28.962; 28.962;
    28.880;
    28.560; 28.070; 26.920; 26.660; 26.500; 25.850; 24.690;
    22.660; 19.940; 17.940; 16.840; 16.170; 16.17];
LR = [-6.5e-3; 0; 1e-3; 2.8e-3; 0; -2.8e-3; -2e-3;
    1.693e-3; 5.00e-3; 1e-2; 2e-2; 1.5e-2; 1e-2; 7e-3; 5e-3; 4e-3;
    3.3e-3; 2.6e-3; 1.7e-3; 1.1e-3; 0];
rho=zeros(layers+1,1);
P=zeros(layers+1,1);
rho0 = Po/(R*To); P(1) = Po; T(1) = To; rho(1) = rho0; 
for i =1:layers
    if ~(LR(i) == 0)
        C1 = 1 + B*( T(i)/LR(i) - Z(i) );
        C2 = C1*go/(R*LR(i));
        C3 = T(i+1)/T(i);
        C4 = C3^(-C2);
        C5 = exp( go*B*(Z(i+1)-Z(i))/(R*LR(i)) );
        P(i + 1) = P(i)*C4*C5;
        C7 = C2 + 1;
        rho(i + 1) = rho(i)*C5*C3^(-C7);
    else
        C8 = -go*(Z(i+1)-Z(i))*(1 - B*(Z(i + 1) + Z(i))/2)/(R*T(i));
        P(i+1) = P(i)*exp(C8); rho(i+1) = rho(i)*exp(C8);
    end
end
for i = 1:21
    if h < Z(i+1)
        if ~(LR(i)== 0)
            C1 = 1 + B*( T(i)/LR(i) - Z(i) );
            TM = T(i) + LR(i)*(h - Z(i));
            C2 = C1*go/(R*LR(i));
            C3 = TM/T(i);
            C4 = C3^(-C2);
            C5 = exp( B*go*(h - Z(i))/(R*LR(i)) );
            PR = P(i)*C4*C5; %Static Pressure (N/m^2)
            C7 = C2 + 1;
            rhoE = C5*rho(i)*C3^(-C7); %Density (kg/m^3)
        else
            TM = T(i);
            C8 = -go*(h - Z(i))*(1 - (h + Z(i))*B/2)/(R*T(i));
            PR = P(i)*exp(C8); %Static Pressure (N/m^2)
            rhoE = rho(i)*exp(C8); %Density (kg/m^3)
        end
        MOL = M(i) + ( M(i+1)-M(i) )*( h - Z(i) )/( Z(i+1) - Z(i) );
        TM = MOL*TM/Mo; %Kinetic Temperature
        asound = sqrt(gamma*R*TM); % Speed of Sound (m/s)
        MU = Beta*TM^1.5/(TM + S); % Dynamic Viscosity Coeff. (N.s/m^2)
        KT = 2.64638e-3*TM^1.5/(TM + 245.4*10^(-12/TM));
        Vm = sqrt(8*R*TM/pi); m = MOL*1e-3/Na; n = rhoE/m;
        F = sqrt(2)*pi*n*sigma^2*Vm;
        L = Vm/F; % Mean free-path (m)
        Mach = vel/asound; % Mach Number
        T0 = TM*(1 + (gamma - 1)*Mach^2/2);
        MU0 = Beta*T0^1.5/(T0 + S);
        RE0 = rhoE*vel*CL/MU0;
        RE = rhoE*vel*CL/MU; % Reynold’s Number
        Kn = L/CL; % Knudsen Number
        Kno = 1.25*sqrt(gamma)*Mach/RE0;
        %flow regime parameter
        if Kn >= 10
            d = 1; % free-molecule flow
        elseif Kn <= 0.01
            d = 2; % continuum flow
        else
            d = 3; % transition flow
        end
        Y = [TM; rhoE; Mach; Kn; asound; d; PR; MU; RE; KT];
        return;
    end
end
end

== matlab function Rocket_test/Subsystem1/Drag_Coeff ==
  data: Alpha_eff input; CD output; Mach input
function CD = Drag_Coeff(Alpha_eff ,Mach)



CD = (Alpha_eff * 0.0035 + 0.21) * (1 + Mach/5.714285);
    return;
end

== matlab function Rocket_test/Subsystem1/X_CP ==
  data: Alpha_eff input; XCP output; Mach input
function XCP = Xcenterpressure(Alpha_eff ,Mach)



XCP = 0.4^(Alpha_eff) * 12 + 18;
    return;
end

== matlab function Rocket_test/Subsystem1/Aerodynamic_forces ==
  data: Q input; Faero output; CD input; CL input
function Faero =  aerodynamic_force(Q, CD, CL)
S_ref=7.14
Faero = -(Q) * S_ref * [CD; 0; CL]
    return;
end

== matlab function Rocket_test/Subsystem1/Dynamic pressure ==
  data: rho input; Q output; v input
function Q = fcn(rho,v)

Q = 0.5*rho*v^2;

== matlab function Rocket_test/ECI to ECEF2/MATLAB Function1 ==
  data: t input; C_IE_t output; Omega_earth input
function C_IE_t=ECI2ECEF(t,Omega_earth)
   C_IE_t =  [cos(Omega_earth*t)     sin(Omega_earth*t)  0;...
             -sin(Omega_earth*t)    cos(Omega_earth*t)  0;...
             0                      0                   1];
end

== matlab function Rocket_test/Subsystem3/Effective AoA ==
  data: v input; aoa_eff output
function aoa_eff = fcn(v)


aoa_eff = atan(sqrt(v(2)^2+v(3)^2)/v(1));
aoa_eff(isnan(aoa_eff))=0;

== matlab function Rocket_test/MATLAB Function ==
  data: alpha input; C_BV output; beta input
function C_BV = body2vel_dcm(alpha,beta)

C_BV= [cos(alpha)*cos(beta) sin(beta) sin(alpha)*cos(beta);...
    -cos(alpha)*sin(beta) cos(beta) -sin(alpha)*sin(beta);...
    -sin(alpha) 0 cos(alpha)]

== matlab function Rocket_test/ECI ot Launch Pad/ECI to ECEF4/MATLAB Function1 ==
  data: t input; C_IE_t output; Omega_earth input
function C_IE_t=ECI2ECEF(t,Omega_earth)
   C_IE_t =  [cos(Omega_earth*t)     sin(Omega_earth*t)  0;...
             -sin(Omega_earth*t)    cos(Omega_earth*t)  0;...
             0                      0                   1];
end

== matlab function Rocket_test/Controller/ECI to ECEF1/MATLAB Function1 ==
  data: t input; C_IE_t output; Omega_earth input
function C_IE_t=ECI2ECEF(t,Omega_earth)
   C_IE_t =  [cos(Omega_earth*t)     sin(Omega_earth*t)  0;...
             -sin(Omega_earth*t)    cos(Omega_earth*t)  0;...
             0                      0                   1];
end

== matlab function Rocket_test/Controller/PYR ==
  data: base input; pitch output; yaw output; roll output
function [pitch,yaw,roll] = PYR(base)
x_vec=base(1:3,1)
z_vec=base(1:3,3)

a=[1 0 0]'
b=[x_vec(1) 0 x_vec(3)]'
pitch=atan2(norm(cross(a,b)), dot(a,b))*sign(-x_vec(3))

Ry=[cos(pitch) 0 sin(pitch); 0 1 0; -sin(pitch) 0 cos(pitch)]
a=Ry*[1 0 0]'
b=x_vec
yaw=atan2(norm(cross(a,b)), dot(a,b))*sign(x_vec(2))

Rz=[cos(yaw) sin(yaw) 0; -sin(yaw) cos(yaw) 0; 0 0 1]
a=Ry*[0 0 1]'
b=Rz'*z_vec
roll=atan2(norm(cross(a,b)), dot(a,b))*sign(b(1))
